simulink model "untitled11"  (R2025a)
settings: Solver=VariableStepAuto  StartTime=0.0  StopTime=15.0  RelTol=1e-3
model workspace (MAT data in the model file):
  I = 5
undefined symbols (not defined in the file or in its folder): g, m, R, v0
settings Model: Creator=rikki  LastModifiedBy=rikki

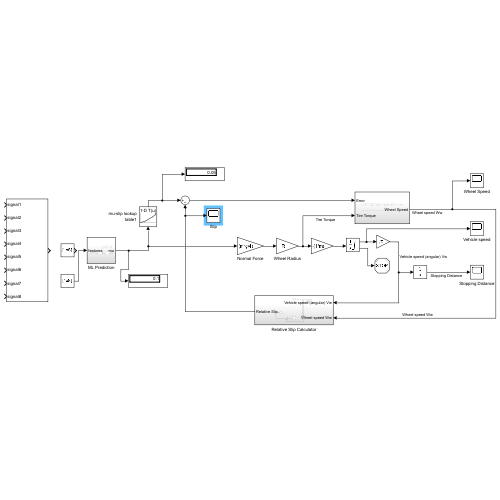
[thumbnail: Simulink's stored preview of the top-level diagram]
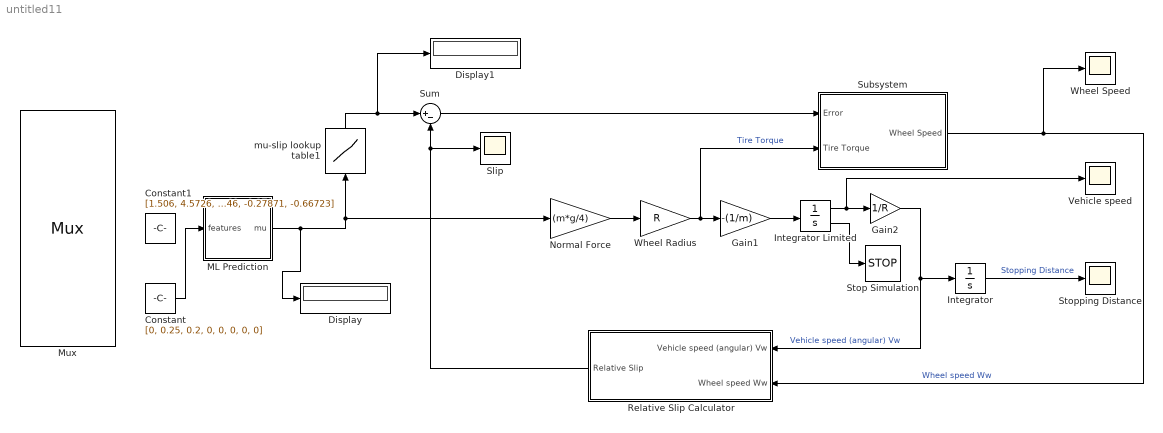
== system untitled11 ==
  Constant : Constant  Value=[0, 0.25, 0.2, 0, 0, 0, 0, 0]  VectorParams1D=off
  Constant1 : Constant  Value=[1.506, 4.5726, 4.7569, 0.29408, -1.3967, 0.28646, -0.27871, -0.66723]  VectorParams1D=off
  Display : Display
  Display1 : Display
  Gain1 : Gain  Gain=-(1/m)
  Gain2 : Gain  Gain=1/R
  Integrator : Integrator
  Integrator Limited : Integrator  InitialCondition=v0  LimitOutput=on  UpperSaturationLimit=1000  LowerSaturationLimit=0  ShowSaturationPort=on
  ML Prediction : Subsystem
  Mux : Mux  Inputs=8
      settings: DisplayOption=signals
  Normal Force : Gain  Gain=(m*g/4)
  Relative Slip Calculator : Subsystem
  "Slip " : Scope
      settings: ActiveDisplayYMinimum=-3.595110523656293  ActiveDisplayYMaximum=3.0181008515479131
  Stop Simulation : Stop
  Stopping Distance : Scope
      settings: ActiveDisplayYMinimum=-4536.5009763227672  ActiveDisplayYMaximum=4911.3287682384989
  Subsystem : Subsystem
  Sum : Sum  Inputs=|+-
  Vehicle speed : Scope
      settings: ActiveDisplayYMinimum=-33.896115950547987  ActiveDisplayYMaximum=98.434444432964568  DataLoggingVariableName=ScopeData3
  Wheel Radius : Gain  Gain=R
  Wheel Speed : Scope
      settings: ActiveDisplayYMinimum=-17.426527734874874  ActiveDisplayYMaximum=90.36656647976028  DataLoggingVariableName=ScopeData2
  mu-slip lookup table1 : Lookup_n-D  NumberOfTableDimensions=1  BreakpointsForDimension1=[0.1,0.4,0.8,0.97,1]  Table=[0.05,0.1,0.2,0.25,0.3]  InternalRulePriority=Speed  RndMeth=Simplest
  wires:
  Integrator/1 -> Stopping Distance/1  "Stopping Distance"
  Integrator Limited/1 -> Vehicle speed/1, Gain2/1
  Gain1/1 -> Integrator Limited/1
  Gain2/1 -> Relative Slip Calculator/1(Vehicle speed (angular) Vw), Integrator/1  "Vehicle speed (angular) Vw"
  Subsystem/1(Wheel Speed) -> Relative Slip Calculator/2(Wheel speed Ww), Wheel Speed/1  "Wheel speed Ww"
  ML Prediction/1(mu) -> Display/1, mu-slip lookup table1/1, Normal Force/1
  Relative Slip Calculator/1(Relative Slip) -> "Slip "/1, Sum/2
  Sum/1 -> Subsystem/1(Error)
  Integrator Limited/2 -> Stop Simulation/1
  Normal Force/1 -> Wheel Radius/1
  Wheel Radius/1 -> Gain1/1, Subsystem/2(Tire Torque)  "Tire Torque"
  mu-slip lookup table1/1 -> Display1/1, Sum/1
  Constant/1 -> ML Prediction/1(features)

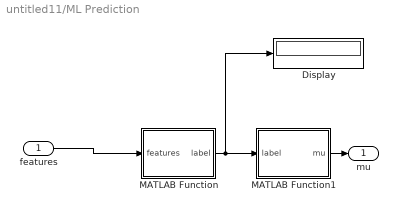
== system untitled11/ML Prediction ==
  features : Inport
  Display : Display
  MATLAB Function : MATLAB Function  TreatAsAtomicUnit=on
  MATLAB Function1 : MATLAB Function  TreatAsAtomicUnit=on
  mu : Outport
  wires:
  MATLAB Function/1(label) -> Display/1, MATLAB Function1/1(label)
  MATLAB Function1/1(mu) -> mu/1
  features/1 -> MATLAB Function/1(features)

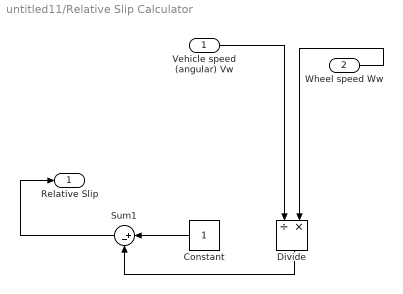
== system untitled11/Relative Slip Calculator ==
  Vehicle speed (angular) Vw : Inport
  Wheel speed Ww : Inport  Port=2
  Constant : Constant
  Divide : Product  Inputs=/*
  Sum1 : Sum  Inputs=|+-
  Relative Slip : Outport  VectorParamsAs1DForOutWhenUnconnected=off
  wires:
  Divide/1 -> Sum1/2
  Sum1/1 -> Relative Slip/1
  Constant/1 -> Sum1/1
  Wheel speed Ww/1 -> Divide/2
  Vehicle speed (angular) Vw/1 -> Divide/1

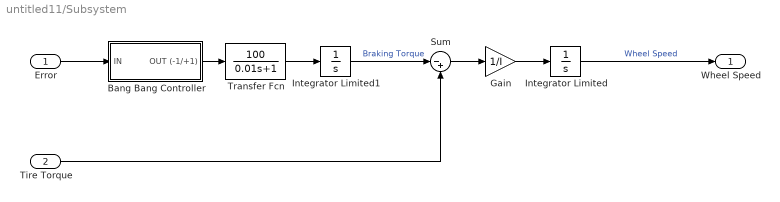
== system untitled11/Subsystem ==
  Error : Inport
  Tire Torque : Inport  Port=2
  Bang Bang Controller : Subsystem
  Gain : Gain  Gain=1/I
  Integrator Limited : Integrator  InitialCondition=v0/R  LimitOutput=on  UpperSaturationLimit=1000  LowerSaturationLimit=0
  Integrator Limited1 : Integrator  LimitOutput=on  UpperSaturationLimit=1500  LowerSaturationLimit=0
  Sum : Sum  Inputs=|-+
  Transfer Fcn : TransferFcn  Numerator=[100]  Denominator=[0.01 1]
  Wheel Speed : Outport  VectorParamsAs1DForOutWhenUnconnected=off
  wires:
  Sum/1 -> Gain/1
  Transfer Fcn/1 -> Integrator Limited1/1
  Gain/1 -> Integrator Limited/1
  Integrator Limited/1 -> Wheel Speed/1  "Wheel Speed"
  Integrator Limited1/1 -> Sum/1  "Braking Torque"
  Bang Bang Controller/1(OUT (-1/+1)) -> Transfer Fcn/1
  Tire Torque/1 -> Sum/2
  Error/1 -> Bang Bang Controller/1(IN)

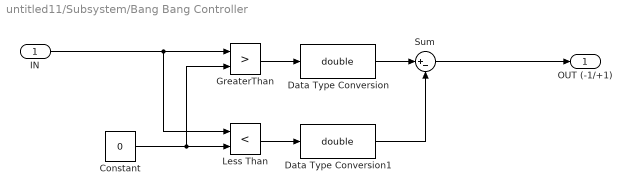
== system untitled11/Subsystem/Bang Bang Controller ==
  IN : Inport
  Constant : Constant  Value=0
  Data Type Conversion : DataTypeConversion  OutDataTypeStr=double  SaturateOnIntegerOverflow=off
  Data Type Conversion1 : DataTypeConversion  OutDataTypeStr=double  SaturateOnIntegerOverflow=off
  GreaterThan : RelationalOperator  Operator=>  OutDataTypeStr=boolean  RndMeth=Simplest  InputSameDT=off
  Less Than : RelationalOperator  Operator=<  OutDataTypeStr=boolean  RndMeth=Simplest  InputSameDT=off
  Sum : Sum  Inputs=|+-
  OUT (-1/+1) : Outport  VectorParamsAs1DForOutWhenUnconnected=off
  wires:
  Sum/1 -> OUT (-1/+1)/1
  Data Type Conversion/1 -> Sum/1
  Constant/1 -> GreaterThan/2, Less Than/2
  IN/1 -> Less Than/1, GreaterThan/1
  Data Type Conversion1/1 -> Sum/2
  GreaterThan/1 -> Data Type Conversion/1
  Less Than/1 -> Data Type Conversion1/1

== matlab function untitled11/ML Prediction/MATLAB Function ==
  data: features input; label output
function label = predictRoadType(features)
%#codegen
persistent model

if isempty(model)
    model = loadLearnerForCoder('roadPredictor');
end

% Create table with correct column names
predictorNames = {'VehicleSpeedInstantaneous', 'LongitudinalAcceleration', ...
                  'VerticalAcceleration', 'MassAirFlow', ...
                  'EngineLoad', 'EngineRPM', ...
                  'ManifoldAbsolutePressure', 'IntakeAirTemperature'};

T = array2table(features, 'VariableNames', predictorNames);

% Predict road surface type
label = predict(model, T);

== matlab function untitled11/ML Prediction/MATLAB Function1 ==
  data: label input; mu output
function mu = getFriction(label)
%#codegen
if label == 0
    mu = 0.8;
elseif label == 1
    mu = 0.4;
else
    mu = 0.1;
end
